simulink model "NLMPC_Monza_simulacion"  (R2023b)
settings: Solver=VariableStepAuto  StartTime=0.0  StopTime=10  RelTol=1e-3
values from neighbouring files (symbols this model uses):
  difficulty = 4    [simulacion_monza_tfm.m]
  Ts = 0.033    [simulacion_monza_tfm.m]
libraries: mpclib x1
settings Model: Creator=christian  LastModifiedBy=lucas
settings SolverCC: AlgebraicLoopSolver=TrustRegion
settings DataIOCC: ReturnWorkspaceOutputs=off
settings DebuggingCC: UnconnectedInputMsg=warning  UnconnectedOutputMsg=warning  UnconnectedLineMsg=warning  ArithmeticOperatorsInVariantConditions=warning
settings ModelReferenceCC: EnableRefExpFcnMdlSchedulingChecks=on
settings SFSimCC: SimUseLocalCustomCode=off  CustomCodeUndefinedFunction=UseInterfaceOnly
settings RTWCC: RTWUseLocalCustomCode=off

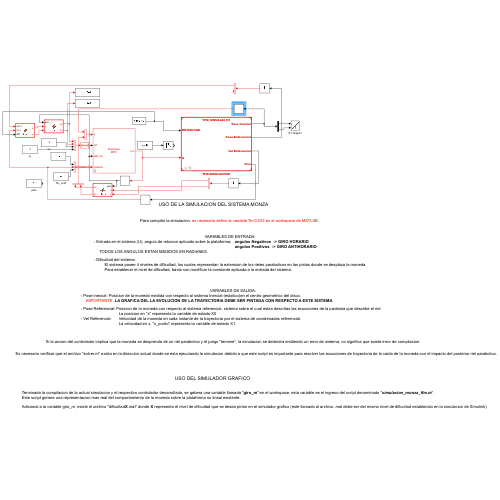
[thumbnail: Simulink's stored preview of the top-level diagram]
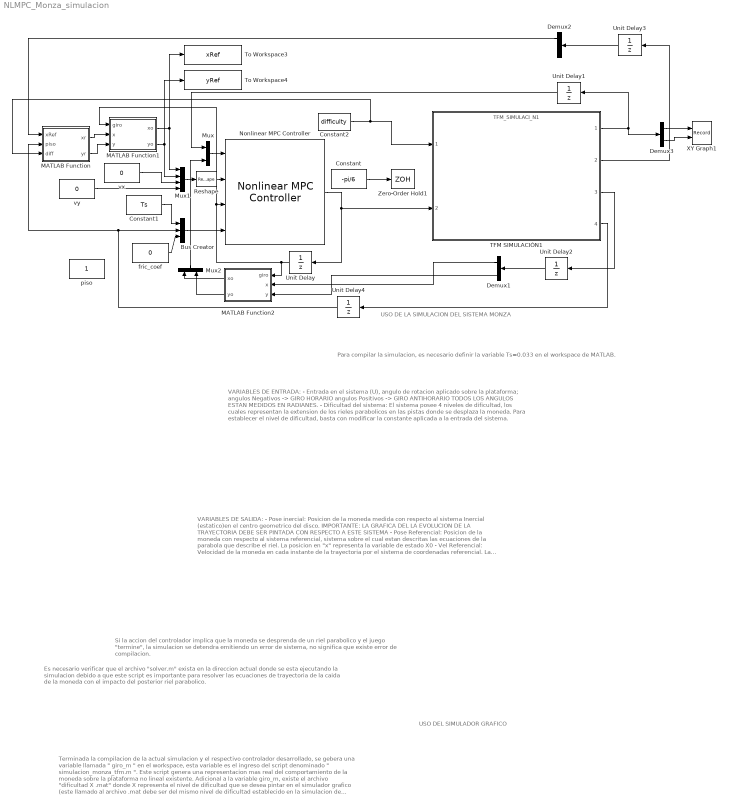
== system NLMPC_Monza_simulacion ==
  note: Es necesario verificar que el archivo "solver.m" exista en la direccion actual donde se esta ejecutando la simulacion debido a que este script es importante para resolver las ecuaciones de trayectoria de la caida de la moneda con el impacto del posterior riel parabolico.
  note: Si la accion del controlador implica que la moneda se desprenda de un riel parabolico y el juego "termine", la simulacion se detendra emitiendo un error de sistema, no significa que existe error de compilacion.
  note: Para compilar la simulacion, es necesario definir la variable Ts=0.033 en el workspace de MATLAB.
  note: VARIABLES DE ENTRADA:
      | - Entrada en el sistema (U), angulo de rotacion aplicado sobre la plataforma; angulos Negativos -> GIRO HORARIO
      | angulos Positivos -> GIRO ANTIHORARIO
      | TODOS LOS ANGULOS ESTAN MEDIDOS EN RADIANES.
      |
      | - Dificultad del sistema:
      | El sistema posee 4 niveles de dificultad, los cuales representan la extension de los rieles parabolicos en las pistas donde se desplaza la moneda.
      | Para establecer el nivel de dificultad, basta con modificar la constante aplicada a la entrada del sistema.
  note: USO DE LA SIMULACION DEL SISTEMA MONZA
  note: VARIABLES DE SALIDA:
      | - Pose inercial: Posicion de la moneda medida con respecto al sistema Inercial (estatico)en el centro geometrico del disco.
      | IMPORTANTE: LA GRAFICA DEL LA EVOLUCION DE LA TRAYECTORIA DEBE SER PINTADA CON RESPECTO A ESTE SISTEMA
      |
      | - Pose Referencial: Posicion de la moneda con respecto al sistema referencial, sistema sobre el cual estan descritas las ecuaciones de la parabola que describe el riel.
      | La posicion en "x" representa la variable de estado X0
      | - Vel Referencial: Velocidad de la moneda en cada instante de la trayectoria por el sistema de coordenadas referencial.
      | La velocidad en x, "x_punto" representa la variable de estado X1.
  note: USO DEL SIMULADOR GRAFICO
  note: Terminada la compilacion de la actual simulacion y el respectivo controlador desarrollado, se gebera una variable llamada " giro_m " en el workspace, esta variable es el ingreso del script denominado " simulacion_monza_tfm.m ".
      | Este script genera una representacion mas real del comportamiento de la moneda sobre la plataforma no lineal existente.
      |
      | Adicional a la variable giro_m, existe el archivo "dificultad X .mat" donde X representa el nivel de dificultad que se desea pintar en el simulador grafico (este llamado al archivo .mat debe ser del mismo nivel de dificultad establecido en la simulacion de Simulink)
  Bus Creator : BusCreator  Inputs=3  OutDataTypeStr=Bus: myBusObject  NonVirtualBus=on
      settings: InheritFromInputs=off
  Constant : Constant  Value=-pi/6
  Constant1 : Constant  Value=Ts
  Constant2 : Constant  Value=difficulty
  Demux1 : Demux  Outputs=2
  Demux2 : Demux  Outputs=2
  Demux3 : Demux  Outputs=2
  MATLAB Function : MATLAB Function  TreatAsAtomicUnit=on
  MATLAB Function1 : MATLAB Function  TreatAsAtomicUnit=on
  MATLAB Function2 : MATLAB Function  TreatAsAtomicUnit=on
  Mux : Mux  Inputs=2
  Mux1 : Mux
  Mux2 : Mux  Inputs=2
  Nonlinear MPC Controller : mpclib/Nonlinear MPC Controller  nlmpcobj=controller  UseObjectTs=on  UseMEX=off  md_enabled=off  mvtarget_enabled=off  param_enabled=on  cost_enabled=off  mvseq_enabled=off  stateseq_enabled=off  ovseq_enabled=off  slack_enabled=off  status_enabled=off  ov_min=off  ov_max=off  mv_min=off  mv_max=off  mvrate_min=off  mvrate_max=off  state_min=off  state_max=off  ov_weight=off  mv_weight=off  mvrate_weight=off  ecr_weight=off  nlp_initialize=off
  Reshape : Reshape  OutputDimensionality=Row vector (2-D)
  TFM SIMULACIÓN1 : ModelReference  ModelNameDialog=TFM_SIMULACI_N1.slx  UsingDefaultArgumentValue=0,0  SimulationMode=Normal  ModelReferenceVersion=13.2  Gain=0.05  Gain2=0.0223
  To Workspace3 : ToWorkspace  VariableName=xRef  SampleTime=Ts*5
  To Workspace4 : ToWorkspace  VariableName=yRef  SampleTime=Ts*5
  Unit Delay{,1..4} (5 alike) : UnitDelay  SampleTime=Ts  HasFrameUpgradeWarning=on
  XY Graph1 : Record  FileSettingsInternal="{\"entries\":[{\"content\":{\"excelSettings\":{\"content\":{},\"type\":\"Streamout.ExcelSettings\"}},\"type\":\"Streamout.FileSettingStorage\",\"uuid\":\"\"}],\"packageUris\":[\"http:\\/\\/schema.mathworks.com\\/mf0\\/streamout_blocks\\/R2020a\"],\"version\":\"1.0\"}"  Layout=[1 1]  SignalsInternal="{\"entries\":[{\"content\":{\"signals\":[{\"content\":{\"blockPath\":[],\"dimensions\":[1],\"domain\":\"\",\"lineColor\":\"#a2142f\",\"plots\":[ 1 ],\"port\":1,\"sid\":[\"\"],\"signalID\":1,\"signalName\":\"Demux3:1\"},\"type\":\"RecordBlkView.Signal\",\"uuid\":\"\"},{\"content\":{\"blockPath\":[],\"dimensions\":[1],\"domain\":\"\",\"lineColor\":\"#139fff\",\"plots\":[ 1 ],\"port\":2,\"sid\":[\"\"],\"signalID\":2,\"signalName\":\"Demux3:2\"},\"type\":\"RecordBlkView.Signal\",\"uuid\":\"\"}]},\"type\":\"RecordBlkView.InputSignals\",\"uuid\":\"\"}],\"packageUris\":[\"http:\\/\\/schema.mathworks.com\\/mf0\\/streamout_blocks\\/R2020a\"],\"version\":\"1.0\"}"  VisualizationBindings="{\"xyplotplugin\":{\"info\":[{\"series\":[{\"bindingParametersList\":[{\"parameter\":\"X-Axis\",\"signalID\":1,\"signalName\":\"Demux3:1\"},{\"parameter\":\"Y-Axis\",\"signalID\":2,\"signalName\":\"Demux3:2\"}],\"seriesID\":0}],\"subplotID\":1}]}}"  CompatibilityTag=XY  st=-1
  Zero-Order Hold1 : ZeroOrderHold  SampleTime=Ts*10
  fric_coef : Constant  Value=0
  piso : Constant
  vx : Constant  Value=0
  vy : Constant  Value=0
  wires:
  Demux3/1 -> XY Graph1/1
  Demux3/2 -> XY Graph1/2
  vy/1 -> Mux1/4
  Constant2/1 -> MATLAB Function/3(diff), TFM SIMULACIÓN1/1
  MATLAB Function1/2(yo) -> To Workspace4/1, Mux1/2
  TFM SIMULACIÓN1/1 -> Demux3/1, Unit Delay1/1
  vx/1 -> Mux1/3
  MATLAB Function1/1(xo) -> To Workspace3/1, Mux1/1
  TFM SIMULACIÓN1/3 -> Unit Delay2/1
  MATLAB Function/1(xr) -> MATLAB Function1/2(x)
  Unit Delay/1 -> MATLAB Function1/1(giro), Nonlinear MPC Controller/3, MATLAB Function2/1(giro)
  MATLAB Function/2(yr) -> MATLAB Function1/3(y)
  Bus Creator/1 -> Nonlinear MPC Controller/4
  Mux/1 -> Nonlinear MPC Controller/1
  fric_coef/1 -> Bus Creator/3
  Nonlinear MPC Controller/1 -> Unit Delay/1, TFM SIMULACIÓN1/2
  Reshape/1 -> Nonlinear MPC Controller/2
  Mux1/1 -> Reshape/1
  Constant/1 -> Zero-Order Hold1/1
  Constant1/1 -> Bus Creator/1
  Unit Delay1/1 -> Mux/1
  Unit Delay2/1 -> Demux1/1
  Mux2/1 -> Mux/2
  Demux1/1 -> MATLAB Function2/2(x)
  Demux1/2 -> MATLAB Function2/3(y)
  MATLAB Function2/1(xo) -> Mux2/1
  MATLAB Function2/2(yo) -> Mux2/2
  Demux2/1 -> MATLAB Function/1(xRef)
  Unit Delay3/1 -> Demux2/1
  TFM SIMULACIÓN1/2 -> Unit Delay3/1
  TFM SIMULACIÓN1/4 -> Unit Delay4/1
  Unit Delay4/1 -> MATLAB Function/2(piso), Bus Creator/2

== matlab function NLMPC_Monza_simulacion/MATLAB Function1 ==
  data: giro input; x input; xo output; y input; yo output
function [xo,yo] = rotate(giro,x,y)
    xo=x*cos(giro)-y*sin(giro);
    yo=x*sin(giro)+y*cos(giro);
end

== matlab function NLMPC_Monza_simulacion/MATLAB Function ==
  data: xRef input; piso input; xr output; diff input; yr output
function [xr, yr] = fcn(xRef,piso,diff)
    if mod(piso,2) == 0
        xRef = xRef - 0.0000001;
    else
        xRef = xRef + 0.0000001;
    end
    switch piso
    case 2
        yRot = -0.54 * (xRef * xRef) + 0.0686;
    case 3
        yRot = -0.54 * (xRef * xRef) + 0.03;
    case 4
        yRot = -0.54 * (xRef * xRef) -0.03;
    case 5
        yRot = -0.54 * (xRef * xRef) - 0.0686;
    case 6
        yRot = -0.54 * (xRef * xRef) - 0.1143;
    case 7
        yRot = -0.54 * (xRef * xRef) - 0.16;
    otherwise
        yRot = -0.54 * (xRef * xRef) + 0.1143;
    end
    switch diff
    case 2
        switch piso
            case 2
                x = -0.04758; y = 0.06799;
            case 3
                x = 0.04969; y = 0.02154;
            case 4
                x = -0.04847; y = -0.02411;
            case 5
                x = 0.04406; y = -0.06961;
            case 6
                x = -0.05409; y = -0.11585;
            case 7
                x = -0.02554; y = -0.16035;
            otherwise
                x = 0.06211; y = 0.11223;
        end
    otherwise
        switch piso
            case 2
                x = 0; y = 0.06857;
            case 3
                x = 0; y = 0.02286;
            case 4
                x = 0; y = -0.02286;
            case 5
                x = 0; y = -0.06857;
            case 6
                x = 0; y = -0.11429;
            case 7
                x = -0.02554; y = -0.16035;
            otherwise
                x = 0; y = 0.11429;
        end
        
    end
    if mod(piso,2) == 0
        if xRef < x
            xr = x; yr = y;
        else
            xr = xRef; yr = yRot;
        end
    else
        if xRef > x
            xr = x; yr = y;
        else
            xr = xRef; yr = yRot;
        end
    end

== matlab function NLMPC_Monza_simulacion/MATLAB Function2 ==
  data: giro input; x input; xo output; y input; yo output
function [xo,yo] = rotate(giro,x,y)
    xo=x*cos(giro)-y*sin(giro);
    yo=x*sin(giro)+y*cos(giro);
end
